simulink subsystem "SlipRateClc"  (R2021b)
settings: Solver=VariableStepAuto  StartTime=0.0  StopTime=10.0  RelTol=1e-3
settings Model: Creator=tsuyoshi  LastModifiedBy=tsuyoshi

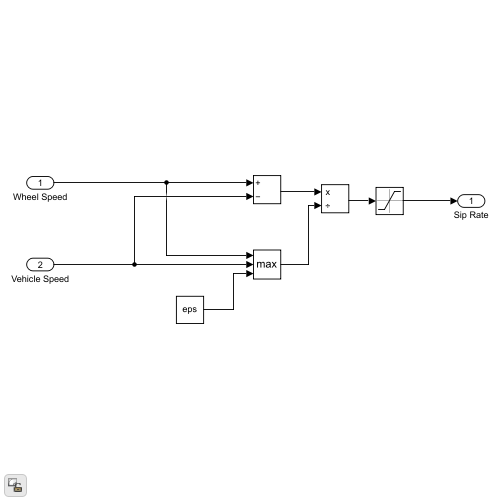
[thumbnail: Simulink's stored preview of the top-level diagram]
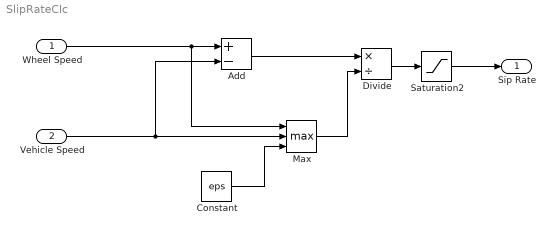
== system SlipRateClc ==
  Wheel Speed : Inport
  Vehicle Speed : Inport  Port=2
  Add : Sum  Inputs=+-
  Constant : Constant  Value=eps
  Divide : Product  Inputs=*/
  Max : MinMax  Function=max  Inputs=3
  Saturation2 : Saturate  UpperLimit=1  LowerLimit=-1
  Sip Rate : Outport  VectorParamsAs1DForOutWhenUnconnected=off
  wires:
  Vehicle Speed/1 -> Max/2, Add/2
  Constant/1 -> Max/3
  Max/1 -> Divide/2
  Divide/1 -> Saturation2/1
  Wheel Speed/1 -> Max/1, Add/1
  Add/1 -> Divide/1
  Saturation2/1 -> Sip Rate/1
